simulink model "aircraft_model_simulink"  (R2022a)
settings: Solver=VariableStepAuto  StartTime=0.0  StopTime=10.0  RelTol=1e-3
values from neighbouring files (symbols this model uses):
  A = [0 1 0 0 0 ... (first row only)    [Aircraft_model.m]    (also in LTR.m = [0 0 -10 0)
  B = [0; 0;0;0;w_a^2]    [Aircraft_model.m]    (also in LTR.m = [0 0; 0 0; 8.533 0; 0 8.533])
  C = eye(5)    [Aircraft_model.m]    (also in LTR.m = [0.5 0.5 0 0)
  C2 = [1 0 0 0 0 ... (first row only)    [Aircraft_model.m]
  D = [0;0;0;0;0]    [Aircraft_model.m]    (also in LTR.m = zeros(2,2))
  D2 = zeros(4,1)    [Aircraft_model.m]
  Gamma = sysd.B    [Aircraft_model.m]    (also in LTR.m)
  K = K_a(:,2:5)    [LTR.m]
  Phi = sysd.A    [Aircraft_model.m]    (also in LTR.m)
  R = 1    [Aircraft_model.m]
undefined symbols (not defined in the file or in its folder): Continuous, Discrete, Kd, Time
libraries: ctrlSharedLib x4, commchan3 x2
settings Model: Creator=mjwhi  LastModifiedBy=mjwhi

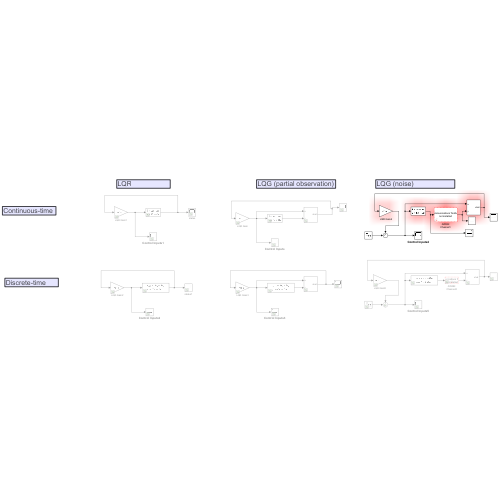
[thumbnail: Simulink's stored preview of the top-level diagram]
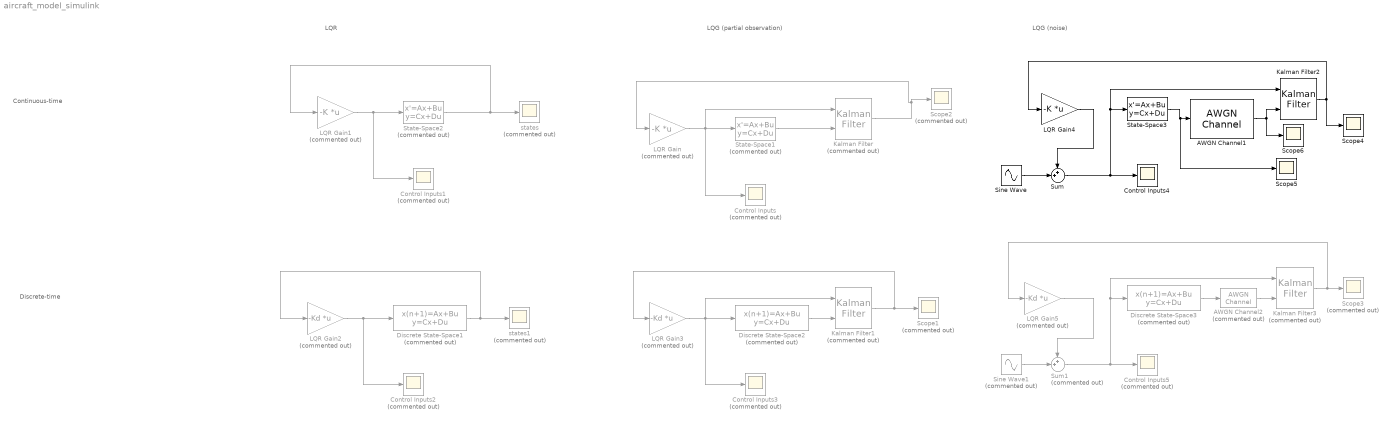
== system aircraft_model_simulink ==
  note: Continuous-time
  note: Discrete-time
  note: LQR
  note: LQG (partial observation)
  note: LQG (noise)
  AWGN Channel1 : commchan3/AWGN Channel  InputProcessing=Columns as channels (frame based)  seed=67  noiseMode="Signal to noise ratio  (SNR)"  EbNodB=10  EsNodB=10  SNRdB=200  bitsPerSym=1  Ps=1  Tsym=1  variance=1
  AWGN Channel2 : commchan3/AWGN Channel  Commented=on  InputProcessing=Columns as channels (frame based)  seed=67  noiseMode="Signal to noise ratio  (SNR)"  EbNodB=10  EsNodB=10  SNRdB=200  bitsPerSym=1  Ps=1  Tsym=1  variance=1
  Control Inputs{,1..3,5} (5 alike) : Scope  Commented=on
  Control Inputs4 : Scope
  Discrete State-Space1 : DiscreteStateSpace  Commented=on  A=Phi  B=Gamma  C=C  D=D  InitialCondition=[0.5 0.5 0.5 0.5 0.5]  SampleTime=-1
  Discrete State-Space2 : DiscreteStateSpace  Commented=on  A=Phi  B=Gamma  C=C2  D=D2  InitialCondition=[0.5;0;0;0;0]  SampleTime=-1
  Discrete State-Space3 : DiscreteStateSpace  Commented=on  A=Phi  B=Gamma  C=C2  D=D2  InitialCondition=[0.5;0;0;0;0]  SampleTime=-1
  Kalman Filter : ctrlSharedLib/Kalman Filter  Commented=on  TimeDomain=Continuous-Time  UseCurrentEstimator=on  ModelSource=Individual A, B, C, D matrices  ModelSourceVariable=ss(0.95,1,1,0,1)  A=A  B=B  C=C2  D=D2  NumberOfStates=1  NumberOfInputs=1  NumberOfOutputs=1  InitialEstimateSource=Dialog  X0=[0 0 0 0 0]  P0=10  UseK=off  UseGH=off  NumberOfProcessNoiseInputs=1  G=1  TimeInvariantG=on  H=0  TimeInvariantH=on  Q=diag([1 0 0 0 0])  TimeInvariantQ=on  R=R  TimeInvariantR=on  N=0  TimeInvariantN=on  AddInputPort=on  AddEnablePort=off  OutputEstimatedY=off  OutputP=off  Ts=-1
  Kalman Filter1 : ctrlSharedLib/Kalman Filter  Commented=on  TimeDomain=Discrete-Time  UseCurrentEstimator=on  ModelSource=Individual A, B, C, D matrices  ModelSourceVariable=ss(0.95,1,1,0,1)  A=Phi  B=Gamma  C=C2  D=D2  NumberOfStates=1  NumberOfInputs=1  NumberOfOutputs=1  InitialEstimateSource=Dialog  X0=[0 0 0 0 0]  P0=10  UseK=off  UseGH=off  NumberOfProcessNoiseInputs=1  G=1  TimeInvariantG=on  H=0  TimeInvariantH=on  Q=diag([1 0 0 0 0])  TimeInvariantQ=on  R=R  TimeInvariantR=on  N=0  TimeInvariantN=on  AddInputPort=on  AddEnablePort=off  OutputEstimatedY=off  OutputP=off  Ts=-1
  Kalman Filter2 : ctrlSharedLib/Kalman Filter  TimeDomain=Continuous-Time  UseCurrentEstimator=on  ModelSource=Individual A, B, C, D matrices  ModelSourceVariable=ss(0.95,1,1,0,1)  A=A  B=B  C=C2  D=D2  NumberOfStates=1  NumberOfInputs=1  NumberOfOutputs=1  InitialEstimateSource=Dialog  X0=[0 0 0 0 0]  P0=10  UseK=off  UseGH=off  NumberOfProcessNoiseInputs=1  G=1  TimeInvariantG=on  H=0  TimeInvariantH=on  Q=diag([1 0 0 0 0])  TimeInvariantQ=on  R=R  TimeInvariantR=on  N=0  TimeInvariantN=on  AddInputPort=on  AddEnablePort=off  OutputEstimatedY=off  OutputP=off  Ts=-1
  Kalman Filter3 : ctrlSharedLib/Kalman Filter  Commented=on  TimeDomain=Discrete-Time  UseCurrentEstimator=on  ModelSource=Individual A, B, C, D matrices  ModelSourceVariable=ss(0.95,1,1,0,1)  A=Phi  B=Gamma  C=C2  D=D2  NumberOfStates=1  NumberOfInputs=1  NumberOfOutputs=1  InitialEstimateSource=Dialog  X0=[0 0 0 0 0]  P0=10  UseK=off  UseGH=off  NumberOfProcessNoiseInputs=1  G=1  TimeInvariantG=on  H=0  TimeInvariantH=on  Q=diag([1 0 0 0 0])  TimeInvariantQ=on  R=R  TimeInvariantR=on  N=0  TimeInvariantN=on  AddInputPort=on  AddEnablePort=off  OutputEstimatedY=off  OutputP=off  Ts=-1
  LQR Gain : Gain  Commented=on  Gain=-K  Multiplication=Matrix(K*u)  SaturateOnIntegerOverflow=on  OutDataTypeStr=Inherit: Same as input  ParamDataTypeStr=Inherit: Same as input
  LQR Gain1 : Gain  Commented=on  Gain=-K  Multiplication=Matrix(K*u)  SaturateOnIntegerOverflow=on  OutDataTypeStr=Inherit: Same as input  ParamDataTypeStr=Inherit: Same as input
  LQR Gain2 : Gain  Commented=on  Gain=-Kd  Multiplication=Matrix(K*u)  SaturateOnIntegerOverflow=on  OutDataTypeStr=Inherit: Same as input  ParamDataTypeStr=Inherit: Same as input
  LQR Gain3 : Gain  Commented=on  Gain=-Kd  Multiplication=Matrix(K*u)  SaturateOnIntegerOverflow=on  OutDataTypeStr=Inherit: Same as input  ParamDataTypeStr=Inherit: Same as input
  LQR Gain4 : Gain  Gain=-K  Multiplication=Matrix(K*u)  SaturateOnIntegerOverflow=on  OutDataTypeStr=Inherit: Same as input  ParamDataTypeStr=Inherit: Same as input
  LQR Gain5 : Gain  Commented=on  Gain=-Kd  Multiplication=Matrix(K*u)  SaturateOnIntegerOverflow=on  OutDataTypeStr=Inherit: Same as input  ParamDataTypeStr=Inherit: Same as input
  Scope1 : Scope  Commented=on
  Scope2 : Scope  Commented=on
  Scope3 : Scope  Commented=on
  Scope4 : Scope
  Scope5 : Scope
  Scope6 : Scope
  Sine Wave : Sin  Frequency=5  SampleTime=0
  Sine Wave1 : Sin  Commented=on  SineType=Sample based  Frequency=5  SampleTime=0.2
  State-Space1 : StateSpace  Commented=on  A=A  B=B  C=C2  D=D2  InitialCondition=[0.5;0;0;0;0]
  State-Space2 : StateSpace  Commented=on  A=A  B=B  C=C  D=D  InitialCondition=[0.5;0;0;0;0]
  State-Space3 : StateSpace  A=A  B=B  C=C2  D=D2  InitialCondition=[0.5;0;0;0;0]
  Sum : Sum  Inputs=++|
  Sum1 : Sum  Commented=on  Inputs=++|
  states : Scope  Commented=on
  states1 : Scope  Commented=on
  wires:
  LQR Gain/1 -> Kalman Filter/1, Control Inputs/1, State-Space1/1
  State-Space1/1 -> Kalman Filter/2
  Kalman Filter/1 -> Scope2/1, LQR Gain/1
  State-Space2/1 -> LQR Gain1/1, states/1
  LQR Gain1/1 -> Control Inputs1/1, State-Space2/1
  LQR Gain2/1 -> Discrete State-Space1/1, Control Inputs2/1
  Discrete State-Space1/1 -> states1/1, LQR Gain2/1
  Kalman Filter1/1 -> Scope1/1, LQR Gain3/1
  Discrete State-Space2/1 -> Kalman Filter1/2
  LQR Gain3/1 -> Discrete State-Space2/1, Control Inputs3/1, Kalman Filter1/1
  Discrete State-Space3/1 -> AWGN Channel2/1
  Kalman Filter3/1 -> LQR Gain5/1, Scope3/1
  Kalman Filter2/1 -> LQR Gain4/1, Scope4/1
  Sine Wave/1 -> Sum/2
  LQR Gain4/1 -> Sum/1
  Sum/1 -> State-Space3/1, Kalman Filter2/1, Control Inputs4/1
  State-Space3/1 -> Scope5/1, AWGN Channel1/1
  AWGN Channel1/1 -> Kalman Filter2/2, Scope6/1
  Sine Wave1/1 -> Sum1/2
  LQR Gain5/1 -> Sum1/1
  Sum1/1 -> Control Inputs5/1, Discrete State-Space3/1, Kalman Filter3/1
  AWGN Channel2/1 -> Kalman Filter3/2
